simulink model "Bai1"  (R2018a)
settings: Solver=ode5  StartTime=0.0  StopTime=60  FixedStep=0.1  RelTol=1e-3
undefined symbols (not defined in the file): sigbuilder_block
libraries: fuzblock x1
settings Model: Creator=ACER  LastModifiedBy=DELL

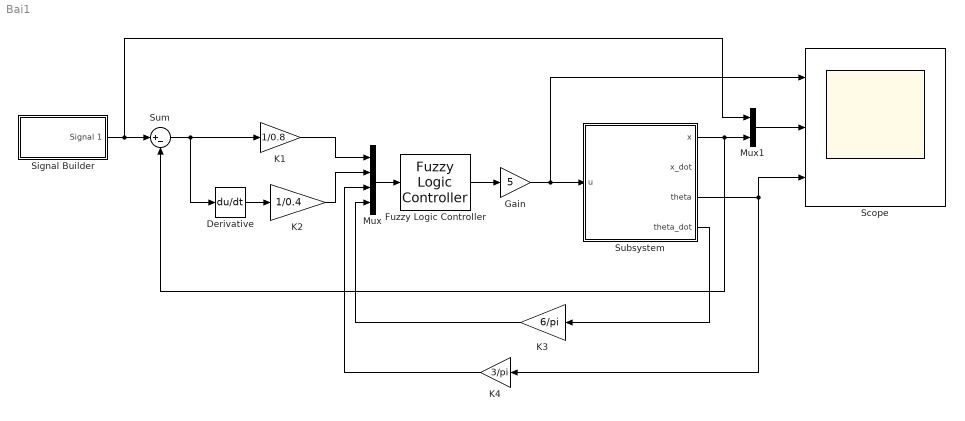
== system Bai1 ==
  Derivative : Derivative
  Fuzzy Logic Controller : fuzblock/Fuzzy Logic  Controller  FIS='fuzzy.fis'  OutputSampleNumber=101  DataType=double  FuzzifiedInputs=off  RuleFiringStrengths=off  RuleOutputs=off  AggregatedOutputs=off  SimulateUsing=Interpreted execution  OutOfRangeInputValueMessage=warning  NoRuleFiredMessage=warning  EmptyOutputFuzzySetMessage=warning
  Gain : Gain  Gain=5
  K1 : Gain  Gain=1/0.8
  K2 : Gain  Gain=1/0.4
  K3 : Gain  Gain=6/pi
  K4 : Gain  Gain=3/pi
  Mux : Mux
  Mux1 : Mux  Inputs=2
  Scope : Scope  NumInputPorts=3
  Signal Builder : Subsystem  Tag=STV Subsys  LoadFcn=sigbuilder_block('load');  StartFcn=sigbuilder_block('start');  StopFcn=sigbuilder_block('stop');  ClipboardFcn=sigbuilder_block('clipboard');  mask(Sigbuilder block){tuvar=[0:10]}
      mask help: Simulink:masks:SigbuilderBlock_MD
      mask init:
      | if ~strcmp(get_param(bdroot(gcbh),'SimulationStatus'),'stopped') tuvar = sigbuilder_block('maskInit'); end
      settings: CopyFcn=sigbuilder_block('copy');  DeleteFcn=sigbuilder_block('delete');  ModelCloseFcn=sigbuilder_block('modelClose');  PreSaveFcn=sigbuilder_block('preSave');  PauseFcn=sigbuilder_block('pause');  ContinueFcn=sigbuilder_block('continue');  NameChangeFcn=sigbuilder_block('namechange');  OpenFcn=sigbuilder_block('open',[5.4 30 1141.2 522.6 ]);  CloseFcn=sigbuilder_block('close');
      mask Display: plot(0, 0, 100, 100,[2, 2, 32, 32, 2], [68, 8, 8, 68, 68],[32, 2], [38, 38], [32, 19, 2],[53, 60, 44], [32, 17, 17, 2],[16, 16, 31, 31]);txt = getActiveGroup(gcbh);text(2, 100, txt,'verticalAlignment', 'top');
  Subsystem : Subsystem  mask{m=0.5, M1=2, l=0.6, g=9.81}
      mask prompts: m "khoi luong xe"; M1 "khoi luong vat nang"; l "chieu dai thanh noi"; g "gia toc trong truong"
  Sum : Sum  Inputs=|+-
  wires:
  Signal Builder/1(Signal 1) -> Mux1/1, Sum/1
  Gain/1 -> Scope/1, Subsystem/1(u)
  Fuzzy Logic Controller/1 -> Gain/1
  Mux/1 -> Fuzzy Logic Controller/1
  K1/1 -> Mux/1
  Sum/1 -> Derivative/1, K1/1
  Mux1/1 -> Scope/2
  Subsystem/1(x) -> Sum/2, Mux1/2
  Subsystem/3(theta) -> K4/1, Scope/3
  Subsystem/4(theta_dot) -> K3/1
  K3/1 -> Mux/4
  K4/1 -> Mux/3
  K2/1 -> Mux/2
  Derivative/1 -> K2/1

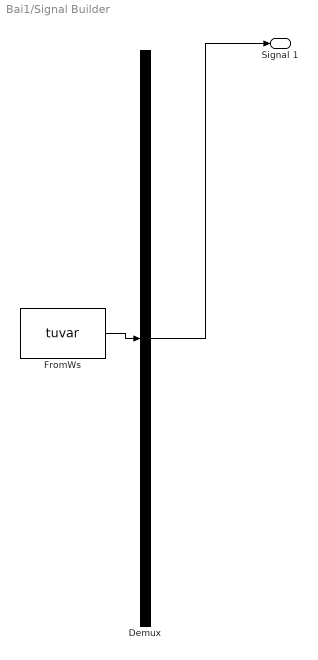
== system Bai1/Signal Builder ==
  Demux : Demux  Tag=STV Demux  Outputs=1
  FromWs : FromWorkspace  Tag=STV FromWs  VariableName=tuvar  SampleTime=0
      SigBuilderData=|
      | common.afterFinalStr = 'Extrapolate'
      | common.sampleTime = 0
      | dataSet.timeRange = [0 60]
      | dataSet.name = 'Group 1'
      | sbobj.Groups.Name = 'Group 1'
      | sbobj.Groups.Signals.Name = 'Signal 1'
      | sbobj.Groups.Signals.XData = [0 9.95 9.95 20.05 20.05 30 30 40.05 40.05 50 50 60]
      | sbobj.Groups.Signals.YData = [0.45 0.45 0.2 0.2 0.8 0.8 0.55 0.55 0.1 0.1 0.65 0.65]
      | sbobj.Groups.TimeRange = [0 60]
  Signal 1 : Outport  Tag=STV Outport
  wires:
  Demux/1 -> Signal 1/1
  FromWs/1 -> Demux/1

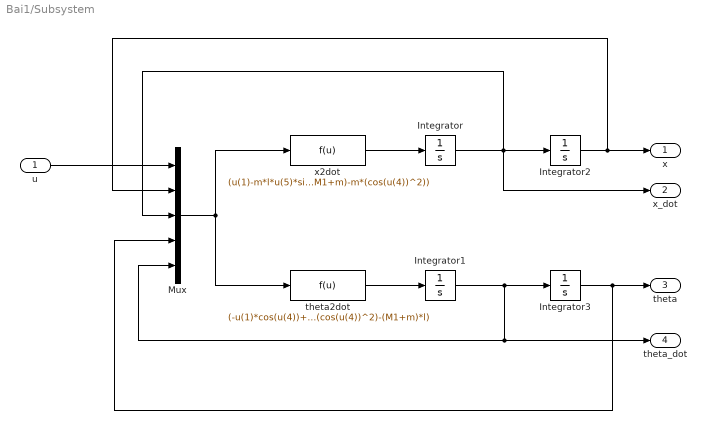
== system Bai1/Subsystem ==
  u : Inport
  Integrator{,1..3} (4 alike) : Integrator
  Mux : Mux  Inputs=5
  theta2dot : Fcn  Expr=(-u(1)*cos(u(4))+m*g*u(5)^2*sin(u(4))*cos(u(4))+(M1+m)*(g*sin(u(4))))/(m*l*(cos(u(4))^2)-(M1+m)*l)
  x2dot : Fcn  Expr=(u(1)-m*l*u(5)*sin(u(4))-m*g*sin(u(4))*cos(u(4)))/((M1+m)-m*(cos(u(4))^2))
  x : Outport
  x_dot : Outport  Port=2
  theta : Outport  Port=3
  theta_dot : Outport  Port=4
  wires:
  x2dot/1 -> Integrator/1
  Integrator/1 -> x_dot/1, Mux/3, Integrator2/1
  theta2dot/1 -> Integrator1/1
  u/1 -> Mux/1
  Mux/1 -> x2dot/1, theta2dot/1
  Integrator2/1 -> x/1, Mux/2
  Integrator3/1 -> theta/1, Mux/4
  Integrator1/1 -> Mux/5, theta_dot/1, Integrator3/1
